simulink model "HHP_simulation"  (R2024b)
settings: Solver=ode23s  StartTime=0.0  StopTime=31104000  FixedStep=10  RelTol=2.42524E-1
undefined symbols (not defined in the file or in its folder): Ar, Br, c1, c33, c4, Cd, Cdl, Cr, Cu, Dd, DiameterLastPiece, dl, Dr, Du, gfunction, L1, L10, np, path_carnot, r_Trichter, Rechenradius, T_null, t_start, t_Trichter, Tdown_0, Tearth_anf, Temperature, Tup_0
libraries: carnot x3
settings Model: SimulationMode=accelerator  Creator=mdraihan  LastModifiedBy=mdraihan
settings SolverCC: MaxConsecutiveMinStep=50  SolverJacobianMethodControl=FullPerturbation  ShapePreserveControl=EnableAll  ZeroCrossControl=DisableAll
settings DataIOCC: LimitDataPoints=on  MaxDataPoints=100  SaveFinalState=on  SaveOperatingPoint=on  SaveFormat=Structure  ReturnWorkspaceOutputs=off  LoggingFileName=logsout
settings DebuggingCC: AlgebraicLoopMsg=none
settings RTWCC: GPUComputeCapability=3.5

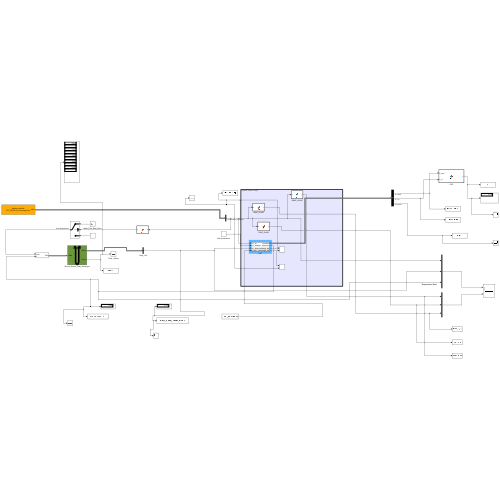
[thumbnail: Simulink's stored preview of the top-level diagram]
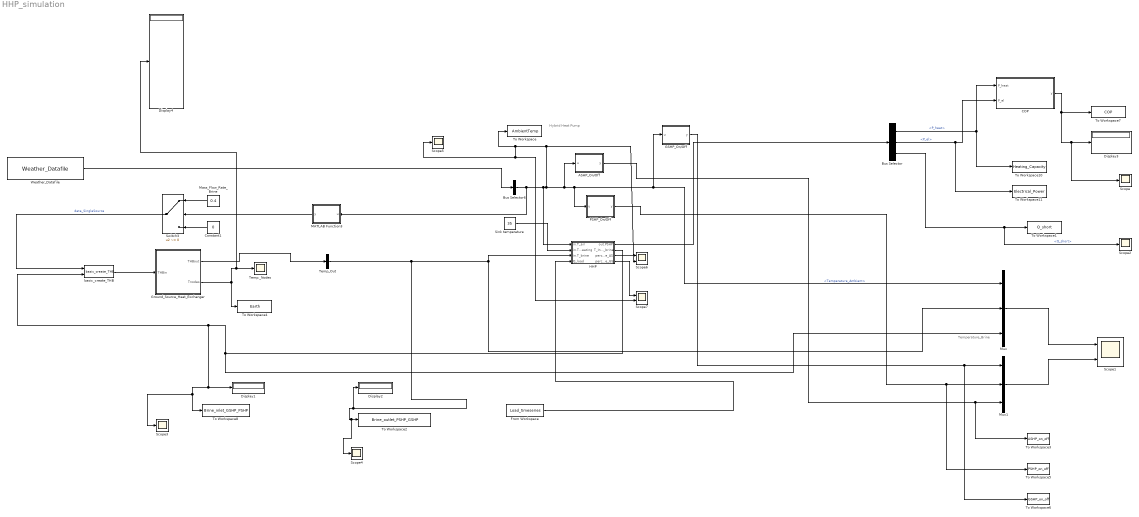
== system HHP_simulation ==
  note: Temperature_Brine
  note: Hybrid Heat Pump
  ASHP_On/Off : MATLAB Function  TreatAsAtomicUnit=on
  Bus Selector : BusSelector  OutputSignals=P_heat,P_el,Q_short
  Bus Selector6 : BusSelector  OutputSignals=Temperature_Ambient
  COP : MATLAB Function  TreatAsAtomicUnit=on
  Constant1 : Constant  Value=0
  Display{1..4} (4 alike) : Display
  From Workspace : FromWorkspace  VariableName=Load_timeseries
  GSHP_On/Off : MATLAB Function  TreatAsAtomicUnit=on
  Ground_Source_Heat_Exchanger : Subsystem  AncestorBlock=carnot/Source/Heat_Exchanger/Ground_Source_Heat_Exchanger  mask(ground source heat exchanger with variable massflow){Jahresmitteltemp_C=10, TGrad=0.025, lambdaErde=2.5, cpErde=1000, rhoErde=2200, lambdaFill=0.81, cpFill=3040, rhoFill=1180, lambda_Sondenrohr=0.48, Massenstrom=0.4, Sondenlaenge=70, B_sondenabstand=5, Sondendurchmesser=0.032, Bohrdurchmesser=0.12, Bu_param=0.12-0.032, Wanddicke_Sondenrohr=0.003, SondenFall=1 probe, DimVert=5, DimRad=10, Gitterfaktor=2.5, LastYear=0, qdot_precalc=10, show=off}
      mask prompts: Jahresmitteltemp_C "Average annual outdoor temperature  in °C"; TGrad "Temperature gradient in K/m, typical 0.025..0.04"; lambdaErde "Thermal conductivity ground in W/m/K"; cpErde "Heat capacity of the ground in J/kg/K"; rhoErde "Denstiy of the ground in kg/m³"; lambdaFill "Thermal conductivity filling in W/m/K"; cpFill "Heat capacity of the filling in J/kg/K"; rhoFill "Denstiy of the filling in kg/m³"; lambda_Sondenrohr "Thermal conductivity of pipe material  in W/m/K"; Massenstrom "Massflow in all ground probes in kg/s"; Sondenlaenge "H: Length of earth probe in m"; B_sondenabstand "B: Probe distance in m (= calculation diameter for single probe)"; Sondendurchmesser "Outer diameter of tube in m"; Bohrdurchmesser "Diameter of drilled hole in m"; Bu_param "Shank spacing in m (must be < borehole diameter)"; Wanddicke_Sondenrohr "Thickness of pipe wall in m"; SondenFall "Field geometry"; DimVert "No. of vertical nodes (typical 5, minimum 2)"; DimRad "No. of horizontal (radial) nodes (typical 10, minimum 3)"; Gitterfaktor "grid factor (typical 2.5, must be > 1)"; LastYear "Year (no precalculation = 0; steady state = 50)"; qdot_precalc "Extraction power per length in W/m (positive for heat removal)"; show "Display start conditions"
      mask help:
      | The CARNOT EWS model is a transient model for dynamic simulation of borehole heat exchangers or so-called vertical ground heat exchangers. The pipe model is for a double U-tube ground probe.  The model is based on the equations described by [Huber] and has been implemented using the state space model of Matlab/Simulink [Bianchi].
      | In the model the matrices are calculated for every timestep to take a variable massflow into account.
      |  See <Help> for literature.
      mask init:
      | DimAxi = max(DimVert*2,4);
      | DimRad = max(DimRad,3);
      | 
      | [Ad,Bd,Cd,Dd, Au,Bu,Cu,Du, Ad0,Bd0, Au0,Bu0, ...
      |     Ar,Br,Cr,Dr, Cdl, c1, c3, c31, c33, c4, c41, c5, c6, ...
      |     L1, L2, L10, L20, dl, Rechenradius, np, ...
      |     Tearth_anf, T_null, teta_fluid_ini, Tdown_0, Tup_0, ...
      |     Ts_Trichter, t_Trichter, r_Trichter, gfunction, t_start ...
      | ] = ...
      | CarnotCallbacks_EWS(LastYear, Massenstrom, qdot_precalc, ...
      |     SondenFall, B_sondenabstand, Sondenlaenge, Sondendurchmesser, ...
      |     Bohrdurchmesser, Bu_param, Wanddicke_Sondenrohr, ...
      |     Jahresmitteltemp_C, TGrad, ...
      |     lambdaErde, rhoErde, cpErde, ...
      |     lambdaFill, cpFill, rhoFill, lambda_Sondenrohr, ...
      |     DimAxi, DimRad, Gitterfaktor, show);
      mask Help: web(fullfile(path_carnot('help'),'Ground_Source_Heat_Exchanger.html'),'-helpbrowser')
      mask TypeOptions SondenFall: 1 probe | 2 probes B/H = 0.1 | 2 probes B/H = 0.05 | 3x6 probes B/H = 0.1 | 5x10 probes B/H = 0.1
      mask DialogControl ParameterTabVar0 Prompt: Thermal
      mask DialogControl ParameterTabVar01 Prompt: Geometry
      mask DialogControl ParameterTabVar012 Prompt: Calculation
      mask DialogControl Container6 Prompt: Precalculation of the ground temperature
      mask Display:
      | plot(0,10,100,90,[70,30],[80,80], ...
      |     [35,35,43,43,47,52,57,57,66,66,60,60,54,46,40,40,35], ...
      |     [84,87,87,20,13,13,21,87,87,84,84,20,10,10,20,84,84])
  HHP : Subsystem
  MATLAB Function3 : MATLAB Function  TreatAsAtomicUnit=on
  Mass_Flow_Rate_Brine : Constant  Value=0.4
  Mux : Mux  Inputs=3
  Mux1 : Mux  Inputs=3
  PSHP_On/Off : MATLAB Function  TreatAsAtomicUnit=on
  Scope{,2..5} (5 alike) : Scope
  Scope1 : Scope  NumInputPorts=2
  Scope6 : Scope  NumInputPorts=2
  Scope7 : Scope  NumInputPorts=2
  Sink temperature : Constant  Value=35
  Switch3 : Switch  Criteria=u2 ~= 0  SaturateOnIntegerOverflow=off
  Temp._Nodes : Scope
  Temp_Out : BusSelector  OutputSignals=Temperature  OutputAsBus=on
  To Workspace : ToWorkspace  VariableName=AmbientTemp  SaveFormat=Structure With Time  SampleTime=-1
  To Workspace1 : ToWorkspace  VariableName=Q_short  SaveFormat=Structure With Time  SampleTime=-1
  To Workspace10 : ToWorkspace  VariableName=Heating_Capacity  SaveFormat=Structure With Time  SampleTime=-1
  To Workspace11 : ToWorkspace  VariableName=Electrical_Power  SaveFormat=Structure With Time  SampleTime=-1
  To Workspace2 : ToWorkspace  VariableName=Brine_outlet_PSHP_GSHP  SaveFormat=Structure With Time  SampleTime=-1
      settings: Save2DSignal=2-D array (concatenate along first dimension)
  To Workspace3 : ToWorkspace  VariableName=ASHP_on_off  SaveFormat=Timeseries  SampleTime=-1
  To Workspace4 : ToWorkspace  VariableName=Earth  SaveFormat=Structure With Time  SampleTime=-1
      settings: Save2DSignal=2-D array (concatenate along first dimension)
  To Workspace5 : ToWorkspace  VariableName=PSHP_on_off  SaveFormat=Timeseries  SampleTime=-1
  To Workspace6 : ToWorkspace  VariableName=GSHP_on_off  SaveFormat=Timeseries  SampleTime=-1
  To Workspace7 : ToWorkspace  VariableName=COP  SampleTime=-1
      settings: Save2DSignal=2-D array (concatenate along first dimension)
  To Workspace8 : ToWorkspace  VariableName=Brine_inlet_GSHP_PSHP  SaveFormat=Structure With Time  SampleTime=-1
  Weather_Datafile : carnot/Weather/Weather_Datafile  PathName=path_carnot('data')  FileName='DE_TRY2010_04_averageYear.mat'  UserParam=off  VariableName=DE_TRY2010_04_averageYear  t_sample=3600
      settings: SourceProductName=Carnot
  basic_create_THB : carnot/Basic/Hydraulics/basic_create_THB  p=2e5  fluid=Water  mix=0  mix2=0  mix3=0  dia=0.03  hgt=0  mID=No Pressure Drop
      settings: SourceProductName=Carnot
  wires:
  Bus Selector/2 -> To Workspace11/1, COP/2(P_el)  "<P_el>"
  HHP/1(out.PSHP) -> Bus Selector/1
  Bus Selector/1 -> COP/1(P_heat), To Workspace10/1  "<P_heat>"
  Switch3/1 -> basic_create_THB/1  "data_SingleSource"
  Bus Selector6/1 -> Scope5/1, Scope7/2, To Workspace/1, Scope6/2, ASHP_On/Off/1(u), PSHP_On/Off/1(u), Mux/1, GSHP_On/Off/1(u), HHP/1(in.T_air), MATLAB Function3/1(u)  "<Temperature_Ambient>"
  Ground_Source_Heat_Exchanger/1(THBout) -> Temp_Out/1
  MATLAB Function3/1(y) -> Switch3/2
  Mass_Flow_Rate_Brine/1 -> Switch3/1
  GSHP_On/Off/1(y) -> To Workspace6/1, Mux1/1
  Mux/1 -> Scope1/1
  Sink temperature/1 -> HHP/2(in.T_heating)
  Weather_Datafile/1 -> Bus Selector6/1
  Constant1/1 -> Switch3/3
  HHP/2(T_Inlet_brine) -> Scope3/1, To Workspace8/1, Display1/1, basic_create_THB/2, Mux/3
  basic_create_THB/1 -> Ground_Source_Heat_Exchanger/1(THBin)
  Ground_Source_Heat_Exchanger/2(Tnodes) -> To Workspace4/1, Temp._Nodes/1, Display4/1
  COP/1(y) -> To Workspace7/1, Scope/1, Display3/1
  ASHP_On/Off/1(y) -> To Workspace3/1, Mux1/3
  From Workspace/1 -> HHP/4(Q_load)
  Mux1/1 -> Scope1/2
  Bus Selector/3 -> Scope2/1, To Workspace1/1  "<Q_short>"
  Temp_Out/1 -> Display2/1, Scope4/1, To Workspace2/1, Mux/2, HHP/3(in.T_brine)
  PSHP_On/Off/1(y) -> To Workspace5/1, Mux1/2
  HHP/3(percentage_AS) -> Scope6/1
  HHP/4(percentage_GS) -> Scope7/1

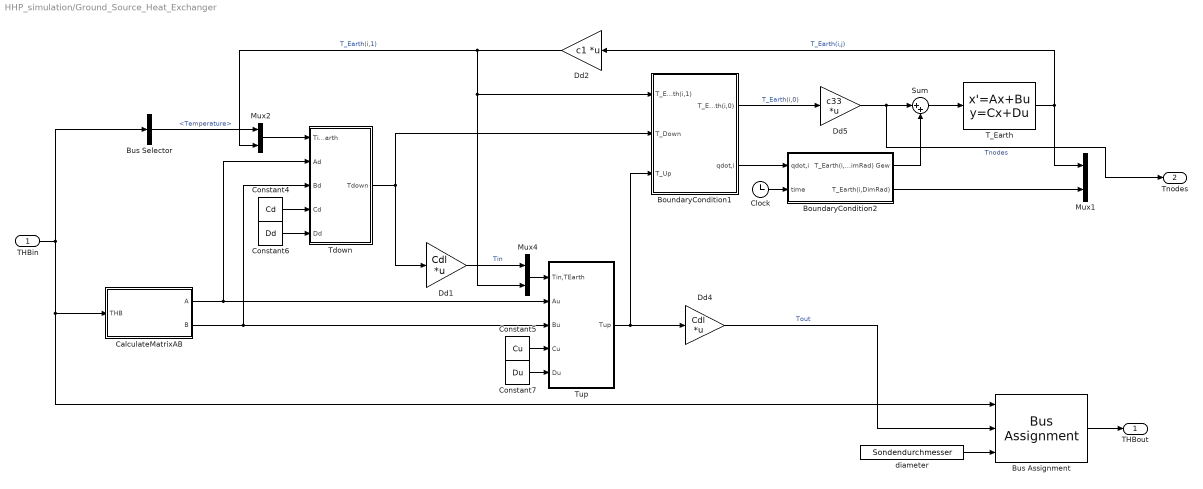
== system HHP_simulation/Ground_Source_Heat_Exchanger ==
  THBin : Inport
  BoundaryCondition1 : Subsystem
  BoundaryCondition2 : Subsystem
  Bus Assignment : BusAssignment  AssignedSignals=Temperature,DiameterLastPiece
  Bus Selector : BusSelector  OutputSignals=Temperature
  CalculateMatrixAB : Subsystem
  Clock : Clock
  Constant4 : Constant  Value=Cd
  Constant5 : Constant  Value=Cu
  Constant6 : Constant  Value=Dd
  Constant7 : Constant  Value=Du
  Dd1 : Gain  Gain=Cdl  Multiplication=Matrix(K*u)  SaturateOnIntegerOverflow=on  OutDataTypeStr=Inherit: Same as input  ParamDataTypeStr=Inherit: Same as input
  Dd2 : Gain  Gain=c1  Multiplication=Matrix(K*u)  SaturateOnIntegerOverflow=on  OutDataTypeStr=Inherit: Same as input  ParamDataTypeStr=Inherit: Same as input
  Dd4 : Gain  Gain=Cdl  Multiplication=Matrix(K*u) (u vector)  SaturateOnIntegerOverflow=on  OutDataTypeStr=Inherit: Same as input  ParamDataTypeStr=Inherit: Same as input
  Dd5 : Gain  Gain=c33  Multiplication=Matrix(K*u) (u vector)  SaturateOnIntegerOverflow=on  OutDataTypeStr=Inherit: Same as input  ParamDataTypeStr=Inherit: Same as input
  Mux1 : Mux  Inputs=2
  Mux2 : Mux  Inputs=2
  Mux4 : Mux  Inputs=2
  Sum : Sum  Inputs=|++  InputSameDT=on  SaturateOnIntegerOverflow=on  OutDataTypeStr=Inherit: Same as first input
  T_Earth : StateSpace  A=Ar  B=Br  C=Cr  D=Dr  InitialCondition=Tearth_anf(:)
  Tdown : Subsystem
  Tup : Subsystem
  diameter : Constant  Value=Sondendurchmesser
  THBout : Outport  VectorParamsAs1DForOutWhenUnconnected=off
  Tnodes : Outport  Port=2  VectorParamsAs1DForOutWhenUnconnected=off
  wires:
  CalculateMatrixAB/2(B) -> Tup/3(Bu), Tdown/3(Bd)
  CalculateMatrixAB/1(A) -> Tup/2(Au), Tdown/2(Ad)
  BoundaryCondition1/2(qdot,i) -> BoundaryCondition2/1(qdot,i)
  Dd4/1 -> Bus Assignment/2  "Tout"
  Bus Assignment/1 -> THBout/1
  diameter/1 -> Bus Assignment/3
  THBin/1 -> CalculateMatrixAB/1(THB), Bus Assignment/1, Bus Selector/1
  BoundaryCondition2/2(T_Earth(i,DimRad)) -> Mux1/2
  Dd2/1 -> Mux4/2, BoundaryCondition1/1(T_Earth(i,1)), Mux2/2  "T_Earth(i,1)"
  BoundaryCondition1/1(T_Earth(i,0)) -> Dd5/1  "T_Earth(i,0)"
  Sum/1 -> T_Earth/1
  BoundaryCondition2/1(T_Earth(i,DimRad) Gew) -> Sum/2
  Tup/1(Tup) -> Dd4/1, BoundaryCondition1/3(T_Up)
  T_Earth/1 -> Dd2/1, Mux1/1  "T_Earth(i,j)"
  Dd1/1 -> Mux4/1  "Tin"
  Mux4/1 -> Tup/1(Tin,TEarth)
  Mux2/1 -> Tdown/1(Tin,TEarth)
  Tdown/1(Tdown) -> Dd1/1, BoundaryCondition1/2(T_Down)
  Constant4/1 -> Tdown/4(Cd)
  Constant6/1 -> Tdown/5(Dd)
  Constant7/1 -> Tup/5(Du)
  Constant5/1 -> Tup/4(Cu)
  Bus Selector/1 -> Mux2/1  "<Temperature>"
  Clock/1 -> BoundaryCondition2/2(time)
  Dd5/1 -> Tnodes/1, Sum/1  "Tnodes"

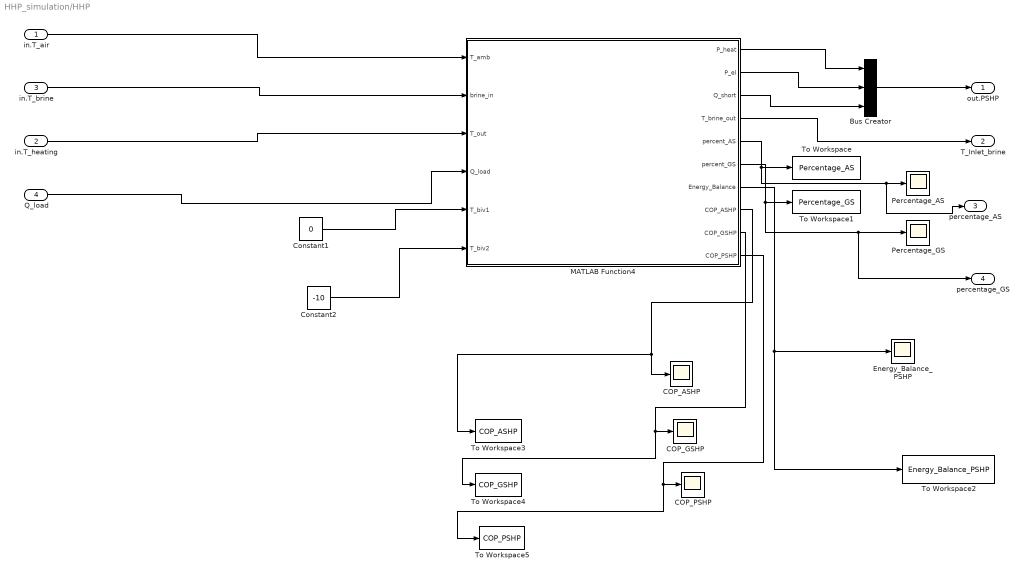
== system HHP_simulation/HHP ==
  in.T_air : Inport
  in.T_heating : Inport  Port=2
  in.T_brine : Inport  Port=3
  Q_load : Inport  Port=4
  Bus Creator : BusCreator  Inputs=3
  COP_ASHP : Scope
  COP_GSHP : Scope
  COP_PSHP : Scope
  Constant1 : Constant  Value=0
  Constant2 : Constant  Value=-10
  Energy_Balance_PSHP : Scope
  MATLAB Function4 : MATLAB Function  TreatAsAtomicUnit=on
  Percentage_AS : Scope
  Percentage_GS : Scope
  To Workspace : ToWorkspace  VariableName=Percentage_AS  SaveFormat=Structure  SampleTime=-1
  To Workspace1 : ToWorkspace  VariableName=Percentage_GS  SaveFormat=Structure  SampleTime=-1
  To Workspace2 : ToWorkspace  VariableName=Energy_Balance_PSHP  SaveFormat=Structure  SampleTime=-1
  To Workspace3 : ToWorkspace  VariableName=COP_ASHP  SaveFormat=Structure  SampleTime=-1
  To Workspace4 : ToWorkspace  VariableName=COP_GSHP  SaveFormat=Structure  SampleTime=-1
  To Workspace5 : ToWorkspace  VariableName=COP_PSHP  SaveFormat=Structure  SampleTime=-1
  out.PSHP : Outport
  T_Inlet_brine : Outport  Port=2
  percentage_AS : Outport  Port=3
  percentage_GS : Outport  Port=4
  wires:
  in.T_air/1 -> MATLAB Function4/1(T_amb)
  in.T_heating/1 -> MATLAB Function4/3(T_out)
  in.T_brine/1 -> MATLAB Function4/2(brine_in)
  Q_load/1 -> MATLAB Function4/4(Q_load)
  MATLAB Function4/4(T_brine_out) -> T_Inlet_brine/1
  MATLAB Function4/2(P_el) -> Bus Creator/2
  MATLAB Function4/1(P_heat) -> Bus Creator/1
  MATLAB Function4/3(Q_short) -> Bus Creator/3
  Bus Creator/1 -> out.PSHP/1
  MATLAB Function4/5(percent_AS) -> percentage_AS/1, Percentage_AS/1, To Workspace/1
  MATLAB Function4/6(percent_GS) -> percentage_GS/1, Percentage_GS/1, To Workspace1/1
  MATLAB Function4/7(Energy_Balance) -> To Workspace2/1, Energy_Balance_PSHP/1
  MATLAB Function4/8(COP_ASHP) -> To Workspace3/1, COP_ASHP/1
  MATLAB Function4/9(COP_GSHP) -> To Workspace4/1, COP_GSHP/1
  MATLAB Function4/10(COP_PSHP) -> To Workspace5/1, COP_PSHP/1
  Constant1/1 -> MATLAB Function4/5(T_biv1)
  Constant2/1 -> MATLAB Function4/6(T_biv2)

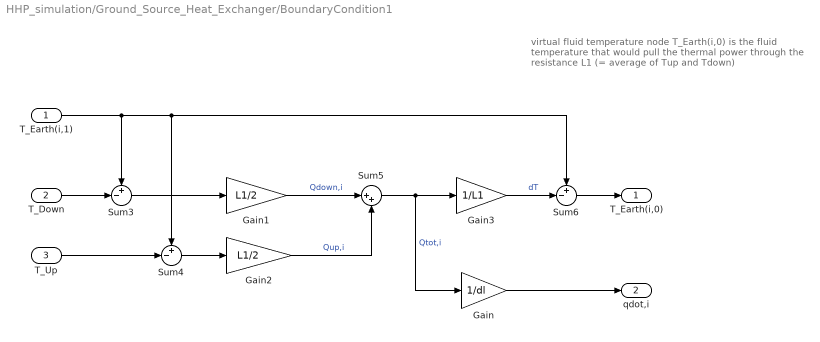
== system HHP_simulation/Ground_Source_Heat_Exchanger/BoundaryCondition1 ==
  note: virtual fluid temperature node T_Earth(i,0) is the
      | fluid temperature that would pull the thermal
      | power through the resistance L1 (= average of
      | Tup and Tdown)
  T_Earth(i,1) : Inport
  T_Down : Inport  Port=2
  T_Up : Inport  Port=3
  Gain : Gain  Gain=1/dl
  Gain1 : Gain  Gain=L1/2  SaturateOnIntegerOverflow=on  OutDataTypeStr=Inherit: Same as input  ParamDataTypeStr=Inherit: Same as input
  Gain2 : Gain  Gain=L1/2  SaturateOnIntegerOverflow=on  OutDataTypeStr=Inherit: Same as input  ParamDataTypeStr=Inherit: Same as input
  Gain3 : Gain  Gain=1/L1  SaturateOnIntegerOverflow=on  OutDataTypeStr=Inherit: Same as input  ParamDataTypeStr=Inherit: Same as input
  Sum3 : Sum  Inputs=+-|  InputSameDT=on  SaturateOnIntegerOverflow=on  OutDataTypeStr=Inherit: Same as first input
  Sum4 : Sum  Inputs=+-|  InputSameDT=on  SaturateOnIntegerOverflow=on  OutDataTypeStr=Inherit: Same as first input
  Sum5 : Sum  Inputs=|++  InputSameDT=on  SaturateOnIntegerOverflow=on  OutDataTypeStr=Inherit: Same as first input
  Sum6 : Sum  Inputs=+-|  InputSameDT=on  SaturateOnIntegerOverflow=on  OutDataTypeStr=Inherit: Same as first input
  T_Earth(i,0) : Outport  VectorParamsAs1DForOutWhenUnconnected=off
  qdot,i : Outport  Port=2  VectorParamsAs1DForOutWhenUnconnected=off
  wires:
  Gain/1 -> qdot,i/1
  Sum6/1 -> T_Earth(i,0)/1
  T_Earth(i,1)/1 -> Sum6/1, Sum4/1, Sum3/1
  Gain3/1 -> Sum6/2  "dT"
  Sum5/1 -> Gain/1, Gain3/1  "Qtot,i"
  Gain2/1 -> Sum5/2  "Qup,i"
  Gain1/1 -> Sum5/1  "Qdown,i"
  Sum4/1 -> Gain2/1
  Sum3/1 -> Gain1/1
  T_Down/1 -> Sum3/2
  T_Up/1 -> Sum4/2

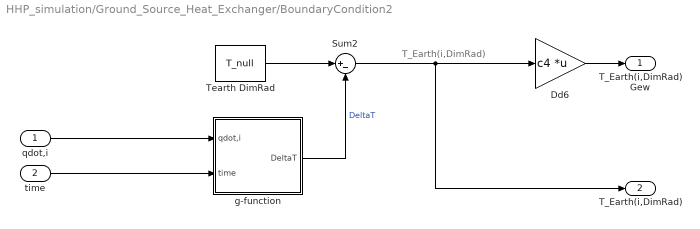
== system HHP_simulation/Ground_Source_Heat_Exchanger/BoundaryCondition2 ==
  note: T_Earth(i,DimRad)
  qdot,i : Inport
  time : Inport  Port=2
  Dd6 : Gain  Gain=c4  Multiplication=Matrix(K*u)  SaturateOnIntegerOverflow=on  OutDataTypeStr=Inherit: Same as input  ParamDataTypeStr=Inherit: Same as input
  Sum2 : Sum  Inputs=|+-  InputSameDT=on  SaturateOnIntegerOverflow=on  OutDataTypeStr=Inherit: Same as first input
  Tearth DimRad : Constant  Value=T_null  VectorParams1D=off
  g-function : Subsystem
  T_Earth(i,DimRad) Gew : Outport  VectorParamsAs1DForOutWhenUnconnected=off
  T_Earth(i,DimRad) : Outport  Port=2  VectorParamsAs1DForOutWhenUnconnected=off
  wires:
  Sum2/1 -> Dd6/1, T_Earth(i,DimRad)/1
  Tearth DimRad/1 -> Sum2/1
  qdot,i/1 -> g-function/1(qdot,i)
  Dd6/1 -> T_Earth(i,DimRad) Gew/1
  g-function/1(DeltaT) -> Sum2/2  "DeltaT"
  time/1 -> g-function/2(time)

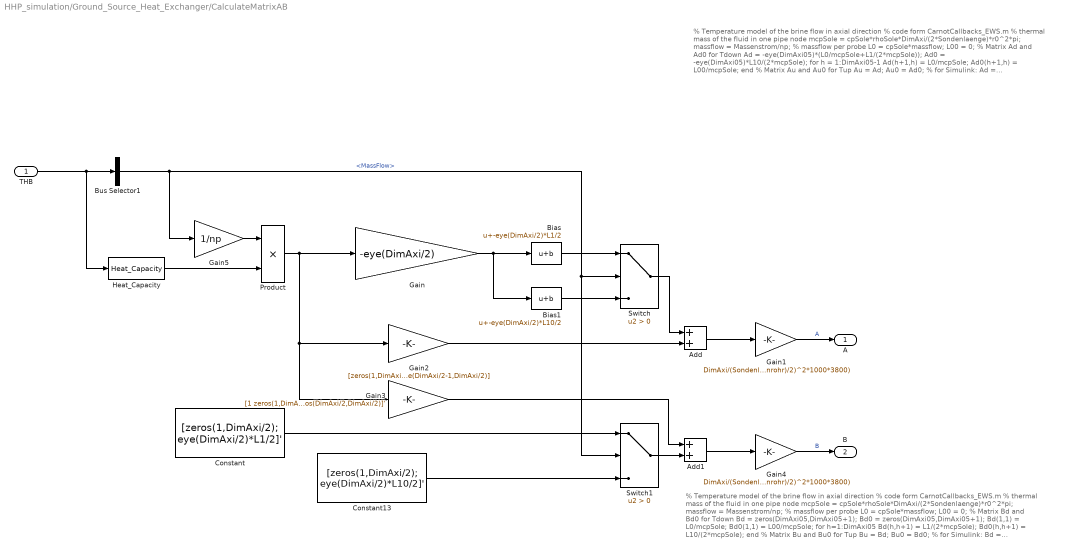
== system HHP_simulation/Ground_Source_Heat_Exchanger/CalculateMatrixAB ==
  note: % Temperature model of the brine flow in axial direction
      | % code form CarnotCallbacks_EWS.m
      | % thermal mass of the fluid in one pipe node
      | mcpSole = cpSole*rhoSole*DimAxi/(2*Sondenlaenge)*r0^2*pi;
      | massflow = Massenstrom/np; % massflow per probe
      | L0 = cpSole*massflow;
      | L00 = 0;
      | % Matrix Bd and Bd0 for Tdown
      | Bd = zeros(DimAxi05,DimAxi05+1);
      | Bd0 = zeros(DimAxi05,DimAxi05+1);
      | Bd(1,1) = L0/mcpSole;
      | Bd0(1,1) = L00/mcpSole;
      | for h=1:DimAxi05
      | Bd(h,h+1) = L1/(2*mcpSole);
      | Bd0(h,h+1) = L10/(2*mcpSole);
      | end
      | % Matrix Bu and Bu0 for Tup
      | Bu = Bd;
      | Bu0 = Bd0;
      |
      | % for Simulink:
      | Bd = [zeros(1,DimAxi/2); eye(DimAxi/2)*L1/2]'
      | Bd = Bd + [1 zeros(1,DimAxi/2-1); zeros(DimAxi/2,DimAxi/2)]'
      | Bd = Bd * DimAxi / ...
      | (Sondenlaenge*2*pi*((Sondendurchmesser-Wanddicke_Sondenrohr)/2)^2*1000*3800)
  note: % Temperature model of the brine flow in axial direction
      | % code form CarnotCallbacks_EWS.m
      | % thermal mass of the fluid in one pipe node
      | mcpSole = cpSole*rhoSole*DimAxi/(2*Sondenlaenge)*r0^2*pi;
      | massflow = Massenstrom/np; % massflow per probe
      | L0 = cpSole*massflow;
      | L00 = 0;
      | % Matrix Ad and Ad0 for Tdown
      | Ad = -eye(DimAxi05)*(L0/mcpSole+L1/(2*mcpSole));
      | Ad0 = -eye(DimAxi05)*L10/(2*mcpSole);
      | for h = 1:DimAxi05-1
      | Ad(h+1,h) = L0/mcpSole;
      | Ad0(h+1,h) = L00/mcpSole;
      | end
      | % Matrix Au and Au0 for Tup
      | Au = Ad;
      | Au0 = Ad0;
      |
      | % for Simulink:
      | Ad = -eye(DimAxi05)
      | Ad = Ad - eye(DimAxi/2)*L1/2
      | Ad = Ad + [zeros(1,DimAxi/2); eye(DimAxi/2-1,DimAxi/2)]
      | Ad = Ad * DimAxi / ...
      | (Sondenlaenge*2*pi*((Sondendurchmesser-Wanddicke_Sondenrohr)/2)^2*1000*3800)
  THB : Inport
  Add : Sum
  Add1 : Sum
  Bias : Bias  Bias=-eye(DimAxi/2)*L1/2  SaturateOnIntegerOverflow=off
  Bias1 : Bias  Bias=-eye(DimAxi/2)*L10/2  SaturateOnIntegerOverflow=off
  Bus Selector1 : BusSelector  OutputSignals=MassFlow
  Constant : Constant  Value=[zeros(1,DimAxi/2); eye(DimAxi/2)*L1/2]'  VectorParams1D=off
  Constant13 : Constant  Value=[zeros(1,DimAxi/2); eye(DimAxi/2)*L10/2]'  VectorParams1D=off
  Gain : Gain  Gain=-eye(DimAxi/2)
  Gain1 : Gain  Gain=DimAxi/(Sondenlaenge*2*pi*((Sondendurchmesser-Wanddicke_Sondenrohr)/2)^2*1000*3800)
  Gain2 : Gain  Gain=[zeros(1,DimAxi/2); eye(DimAxi/2-1,DimAxi/2)]
  Gain3 : Gain  Gain=[1 zeros(1,DimAxi/2-1); zeros(DimAxi/2,DimAxi/2)]'
  Gain4 : Gain  Gain=DimAxi/(Sondenlaenge*2*pi*((Sondendurchmesser-Wanddicke_Sondenrohr)/2)^2*1000*3800)
  Gain5 : Gain  Gain=1/np
  Heat_Capacity : carnot/Basic/Material_Properties/Heat_Capacity  VariantControl=CarlibClassic  INPUTARGUMENTS=THB  DEBUGLEVEL=DEBUGLEVEL  MAXTOTALWARNINGS=0  MAXCONSECUTIVEWARNINGS=0  WRITETOFILE=0  FILENAME='errors.txt'
      settings: SourceProductName=Carnot
  Product : Product
  Switch : Switch  Criteria=u2 > Threshold  SaturateOnIntegerOverflow=off  InputSameDT=off
  Switch1 : Switch  Criteria=u2 > Threshold  SaturateOnIntegerOverflow=off  InputSameDT=off
  A : Outport
  B : Outport  Port=2
  wires:
  Gain5/1 -> Product/1
  Gain4/1 -> B/1  "B"
  Gain1/1 -> A/1  "A"
  Gain3/1 -> Add1/1
  Add1/1 -> Gain4/1
  Constant/1 -> Switch1/1
  Heat_Capacity/1 -> Product/2
  Gain2/1 -> Add/2
  Switch/1 -> Add/1
  Constant13/1 -> Switch1/3
  Add/1 -> Gain1/1
  Switch1/1 -> Add1/2
  Bias/1 -> Switch/1
  Product/1 -> Gain/1, Gain2/1, Gain3/1
  Bias1/1 -> Switch/3
  Gain/1 -> Bias/1, Bias1/1
  Bus Selector1/1 -> Gain5/1, Switch1/2, Switch/2  "<MassFlow>"
  THB/1 -> Heat_Capacity/1, Bus Selector1/1

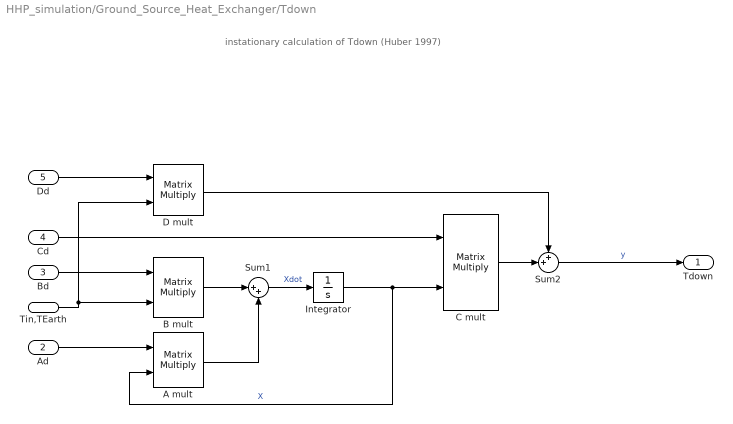
== system HHP_simulation/Ground_Source_Heat_Exchanger/Tdown ==
  note: instationary calculation of Tdown (Huber 1997)
  Tin,TEarth : Inport
  Ad : Inport  Port=2
  Bd : Inport  Port=3
  Cd : Inport  Port=4
  Dd : Inport  Port=5
  A mult : Product  Multiplication=Matrix(*)  RndMeth=Zero
  B mult : Product  Multiplication=Matrix(*)  RndMeth=Zero
  C mult : Product  Multiplication=Matrix(*)  RndMeth=Zero
  D mult : Product  Multiplication=Matrix(*)  RndMeth=Zero
  Integrator : Integrator  InitialCondition=Tdown_0
  Sum1 : Sum  Inputs=|++
  Sum2 : Sum  Inputs=++|
  Tdown : Outport  VectorParamsAs1DForOutWhenUnconnected=off
  wires:
  Sum2/1 -> Tdown/1  "y"
  Tin,TEarth/1 -> B mult/2, D mult/2
  D mult/1 -> Sum2/1
  C mult/1 -> Sum2/2
  B mult/1 -> Sum1/1
  Sum1/1 -> Integrator/1  "Xdot"
  Integrator/1 -> C mult/2, A mult/2  "X"
  A mult/1 -> Sum1/2
  Ad/1 -> A mult/1
  Cd/1 -> C mult/1
  Dd/1 -> D mult/1
  Bd/1 -> B mult/1

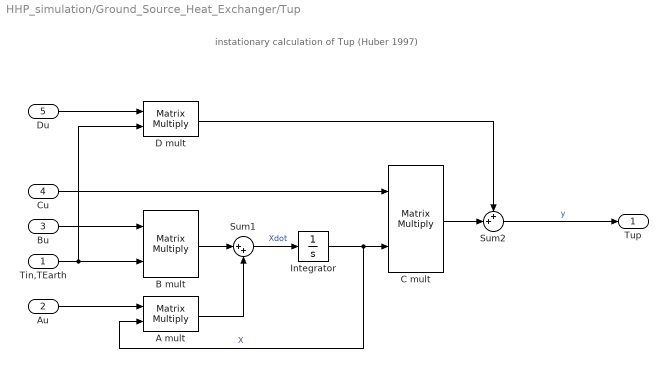
== system HHP_simulation/Ground_Source_Heat_Exchanger/Tup ==
  note: instationary calculation of Tup (Huber 1997)
  Tin,TEarth : Inport
  Au : Inport  Port=2
  Bu : Inport  Port=3
  Cu : Inport  Port=4
  Du : Inport  Port=5
  A mult : Product  Multiplication=Matrix(*)  RndMeth=Zero
  B mult : Product  Multiplication=Matrix(*)  RndMeth=Zero
  C mult : Product  Multiplication=Matrix(*)  RndMeth=Zero
  D mult : Product  Multiplication=Matrix(*)  RndMeth=Zero
  Integrator : Integrator  InitialCondition=Tup_0
  Sum1 : Sum  Inputs=|++
  Sum2 : Sum  Inputs=++|
  Tup : Outport  VectorParamsAs1DForOutWhenUnconnected=off
  wires:
  Sum2/1 -> Tup/1  "y"
  Tin,TEarth/1 -> D mult/2, B mult/2
  D mult/1 -> Sum2/1
  C mult/1 -> Sum2/2
  B mult/1 -> Sum1/1
  Sum1/1 -> Integrator/1  "Xdot"
  Integrator/1 -> A mult/2, C mult/2  "X"
  A mult/1 -> Sum1/2
  Bu/1 -> B mult/1
  Au/1 -> A mult/1
  Cu/1 -> C mult/1
  Du/1 -> D mult/1

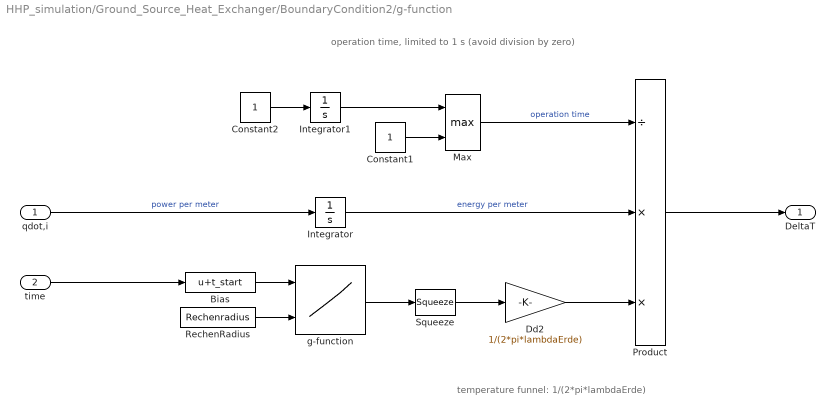
== system HHP_simulation/Ground_Source_Heat_Exchanger/BoundaryCondition2/g-function ==
  note: temperature funnel: 1/(2*pi*lambdaErde)
  note: operation time, limited to 1 s (avoid division by zero)
  qdot,i : Inport
  time : Inport  Port=2
  Bias : Bias  Bias=t_start  SaturateOnIntegerOverflow=off
  Constant1 : Constant
  Constant2 : Constant
  Dd2 : Gain  Gain=1/(2*pi*lambdaErde)  SaturateOnIntegerOverflow=on  OutDataTypeStr=Inherit: Same as input  ParamDataTypeStr=Inherit: Same as input
  Integrator : Integrator
  Integrator1 : Integrator  LowerSaturationLimit=1
  Max : MinMax  Function=max  Inputs=2
  Product : Product  Inputs=/**  InputSameDT=on  RndMeth=Zero  SaturateOnIntegerOverflow=on  OutDataTypeStr=Inherit: Same as first input
  RechenRadius : Constant  Value=Rechenradius  VectorParams1D=off
  Squeeze : Squeeze
  g-function : Lookup_n-D  BreakpointsForDimension1=t_Trichter  BreakpointsForDimension2=r_Trichter  BeginIndexSearchUsingPreviousIndexResult=on  Table=gfunction  InternalRulePriority=Speed  RndMeth=Simplest
      settings: InputPortMap=u0,u1
  DeltaT : Outport  VectorParamsAs1DForOutWhenUnconnected=off
  wires:
  Bias/1 -> g-function/1
  time/1 -> Bias/1
  Constant2/1 -> Integrator1/1
  Max/1 -> Product/1  "operation time"
  Constant1/1 -> Max/2
  Integrator1/1 -> Max/1
  Integrator/1 -> Product/2  "energy per meter"
  Squeeze/1 -> Dd2/1
  qdot,i/1 -> Integrator/1  "power per meter"
  g-function/1 -> Squeeze/1
  Product/1 -> DeltaT/1
  Dd2/1 -> Product/3
  RechenRadius/1 -> g-function/2

== matlab function HHP_simulation/ASHP_On//Off ==
  data: u input; y output
function y = fcn(u)
    % Function to check if the temperature is between 5°C and 13°C
    % Inputs:
    %   u - Temperature (numeric or part of a structure)
    % Outputs:
    %   y - 1 if the temperature is between 5°C and 13°C, 0 otherwise

    % Initialize output
    y = 0;

    % Define the field name (update this if necessary)
    fieldName = 'Temp';

    % Check if input is numeric
    if isnumeric(u)
        % Main logic: check if within range
        if u >= 5 && u <= 13
            y = 1;
        end
    % Check if input is a structure
    elseif isstruct(u)
        % Ensure the structure has the expected field
        if isfield(u, fieldName)
            temp = u.(fieldName); % Extract the temperature field

            % Ensure the extracted value is numeric
            if isnumeric(temp)
                % Main logic: check if within range
                if temp >= 5 && temp <= 13
                    y = 1;
                end
            else
                error('The field "%s" must contain numeric data.', fieldName);
            end
        else
            error('The input structure does not have the field "%s".', fieldName);
        end
    else
        % Handle unsupported input types
        error('Input must be either numeric or a structure with a numeric field "%s".', fieldName);
    end
end

== matlab function HHP_simulation/COP ==
  data: P_heat input; y output; P_el input
function y = fcn(P_heat, P_el)
    % Function to calculate COP based on heating capacity and electrical power.
    % If the heat pump is operating (both P_heat and P_el nonzero), the COP 
    % is computed as P_heat / P_el and forced to be at least 1.
    % If the heat pump is off (either input is 0), the COP is set to 0.
    %
    % Inputs:
    %   P_heat - Heating capacity of the heat pump (W)
    %   P_el   - Electrical power input to the heat pump (W)
    %
    % Outputs:
    %   y - Calculated COP (dimensionless)

    % Handle negative values by treating them as zero.
    if P_heat < 0
        P_heat = 0;
    end
    if P_el < 0
        P_el = 0;
    end

    % Check if the system is off (either P_heat or P_el is zero)
    if (P_heat == 0 || P_el == 0)
        y = 0; % Off condition
    else
        % Calculate COP normally.
        y = P_heat / P_el;
        % If COP is less than 1, set it to 1 (when operating, COP cannot be < 1).
        if y < 1
            y = 1;
        end
    end
end

== matlab function HHP_simulation/HHP/MATLAB Function4 ==
  data: T_amb input; P_heat output; brine_in input; T_out input; Q_load input; P_el output; Q_short output; T_brine_out output; percent_AS output; percent_GS output; Energy_Balance output; COP_ASHP output; COP_GSHP output; COP_PSHP output; T_biv1 input; T_biv2 input
function [P_heat, P_el, Q_short, T_brine_out, percent_AS, percent_GS, Energy_Balance, COP_ASHP, COP_GSHP, COP_PSHP] = hpHeatingPartLoad_Parallel_Final(...
        T_amb, brine_in, T_out, Q_load, T_biv1, T_biv2)
    
    NO_LOAD_THRESHOLD  = 1.0;
    T_amb              = double(T_amb(1));
    brine_in           = double(brine_in(1));
    T_out              = double(T_out(1));
    Q_load             = double(Q_load(1));
    
    if Q_load <= NO_LOAD_THRESHOLD
        P_heat=0; P_el=0; Q_short=Q_load; T_brine_out=brine_in; percent_AS=0;
        percent_GS=0; Energy_Balance=0; COP_ASHP=0; COP_GSHP=0; COP_PSHP=0;
        return;
    end
    
    if T_amb > T_biv1
        Q_AS = Q_load;
        Q_GS = 0;
    elseif T_amb >= T_biv2
        Q_AS = 0;
        Q_GS = Q_load;
    else
        ratio_base = min(max((T_biv2 - T_amb) / 10.0, 0), 1.0);
        ratio_GS = 0.7 + ratio_base * 0.2;
        ratio_AS = 1.0 - ratio_GS;
        Q_AS = Q_load * ratio_AS;
        Q_GS = Q_load * ratio_GS;
    end
    
    m_dot_GS = 0.4;
    delta_T = T_out - brine_in;
    if delta_T > 40, m_dot_GS = 0.6;
    elseif delta_T > 30, m_dot_GS = 0.5;
    else, m_dot_GS = 0.4; end
    if brine_in < 2, m_dot_GS = m_dot_GS * 1.25; end
    
    P_heat_AS=0; P_el_AS=0; Q_short_AS=0;
    P_heat_GS=0; P_el_GS=0; Q_short_GS=0; T_brine_out=brine_in;
    if Q_AS > 0
        [P_heat_AS, P_el_AS, Q_short_AS] = hpHeatingPartLoad_ASHP_Original_PLM(T_amb, T_out, Q_AS);
    end
    if Q_GS > 0
        [P_heat_GS, P_el_GS, Q_short_GS, T_brine_out] = ...
            hpHeatingPartLoad_GSHP_Original_PLM(brine_in, T_out, Q_GS, m_dot_GS);
    end
    
    P_heat  = P_heat_AS + P_heat_GS;
    P_el    = P_el_AS   + P_el_GS;
    Q_short = Q_short_AS + Q_short_GS;
    
    if Q_short > 0 && P_heat > 0
        base_cop = P_heat / P_el;
        stage_up_cop = base_cop * 0.97;
        max_additional_heat = P_heat * 0.15;
        
        P_heat_extra = min(Q_short, max_additional_heat);
        P_el_extra = 0;
        if stage_up_cop > 0
            P_el_extra = P_heat_extra / stage_up_cop;
        end

        P_heat = P_heat + P_heat_extra;
        P_el = P_el + P_el_extra;
        
        Q_short = max(0, Q_load - P_heat);
    end

    if (P_heat > 0) && (P_el > 0)
        if T_amb < T_biv2, max_allowed_COP = 5.0; 
        elseif T_amb > T_biv1, max_allowed_COP = 4.0;
        else, max_allowed_COP = 5.0; end
        current_COP = P_heat / P_el;
        transition_start = max_allowed_COP * 0.75;
        if current_COP > transition_start
            excess_COP = current_COP - transition_start;
            limiting_factor = 1.0 - exp(-3.0 * excess_COP / (max_allowed_COP - transition_start));
            max_excess_allowed = (max_allowed_COP - transition_start) * limiting_factor;
            target_COP = min(transition_start + max_excess_allowed, max_allowed_COP*0.999);
            P_el = P_heat / target_COP;
        end
    end
    
    percent_AS = 0; percent_GS = 0;
    if P_heat > 0
        P_heat_total_no_extra = P_heat_AS + P_heat_GS;
        if P_heat_total_no_extra > 0
             percent_AS = 100 * (P_heat_AS / P_heat_total_no_extra);
             percent_GS = 100 * (P_heat_GS / P_heat_total_no_extra);
        end
    end
    Energy_Balance = P_heat - P_el - ( (P_heat_AS-P_el_AS) + (P_heat_GS-P_el_GS) );

    COP_ASHP = 0; COP_GSHP = 0; COP_PSHP = 0;
    if (P_el > 0) && (P_heat > 0)
        total_COP = P_heat / P_el;
        if T_amb > T_biv1
            temp_range = T_biv1 - T_biv2;
            if temp_range <= 0, temp_range = 12; end
            temp_factor   = max(0.6, min(1.0, (T_amb - T_biv2) / temp_range));
            output_factor = max(0.7, min(1.0, 1 - (T_out - 30)/25 ));
            COP_ASHP = min(total_COP * (temp_factor * output_factor), 4.0 * 0.999);
        elseif T_amb >= T_biv2
            COP_GSHP = total_COP;
        else 
            COP_PSHP = total_COP;
        end
    end
end

function [P_heat, P_el, Q_short] = hpHeatingPartLoad_ASHP_Original_PLM(T_amb, T_out, Q_load)
    if (Q_load <= 0) || (T_amb < -20), P_heat = 0; P_el = 0; Q_short = Q_load; return; end
    T_amb_vec = [-15, -7, 2, 7, 12]; T_out_vec = [30, 35, 40, 45];
    CapacityMatrix = [ 2.47, 2.87, 3.27, 3.64, 4.00; 2.33, 2.73, 3.13, 3.49, 3.85; 2.18, 2.58, 2.98, 3.35, 3.71; 2.04, 2.44, 2.84, 3.20, 3.56 ];
    PowerMatrix = [ 1.20, 0.98, 0.84, 0.78, 0.74; 1.39, 1.14, 0.98, 0.90, 0.82; 1.57, 1.32, 1.07, 0.97, 0.90; 1.74, 1.50, 1.20, 1.12, 1.02 ];
    T_amb_lower_idx=1; for i=1:length(T_amb_vec), if T_amb>=T_amb_vec(i), T_amb_lower_idx=i; end, end
    if T_amb_lower_idx==length(T_amb_vec), T_amb_upper_idx=T_amb_lower_idx; else, T_amb_upper_idx=T_amb_lower_idx+1; end
    T_out_lower_idx=1; for i=1:length(T_out_vec), if T_out>=T_out_vec(i), T_out_lower_idx=i; end, end
    if T_out_lower_idx==length(T_out_vec), T_out_upper_idx=T_out_lower_idx; else, T_out_upper_idx=T_out_lower_idx+1; end
    if (T_amb_lower_idx==T_amb_upper_idx)||(T_out_lower_idx==T_out_upper_idx), Q_rated=CapacityMatrix(T_out_lower_idx,T_amb_lower_idx); P_rated=PowerMatrix(T_out_lower_idx,T_amb_lower_idx);
    else
        x1=T_amb_vec(T_amb_lower_idx);x2=T_amb_vec(T_amb_upper_idx);y1=T_out_vec(T_out_lower_idx);y2=T_out_vec(T_out_upper_idx);
        Q11=CapacityMatrix(T_out_lower_idx,T_amb_lower_idx);Q12=CapacityMatrix(T_out_upper_idx,T_amb_lower_idx);Q21=CapacityMatrix(T_out_lower_idx,T_amb_upper_idx);Q22=CapacityMatrix(T_out_upper_idx,T_amb_upper_idx);
        P11=PowerMatrix(T_out_lower_idx,T_amb_lower_idx);P12=PowerMatrix(T_out_upper_idx,T_amb_lower_idx);P21=PowerMatrix(T_out_lower_idx,T_amb_upper_idx);P22=PowerMatrix(T_out_upper_idx,T_amb_upper_idx);
        wx=(T_amb-x1)/(x2-x1);wy=(T_out-y1)/(y2-y1);
        Q_rated=(1-wx)*(1-wy)*Q11+wx*(1-wy)*Q21+(1-wx)*wy*Q12+wx*wy*Q22;P_rated=(1-wx)*(1-wy)*P11+wx*(1-wy)*P21+(1-wx)*wy*P12+wx*wy*P22;
    end
    Q_rated=max(0.2,Q_rated);P_rated=max(0.1,P_rated);
    PLR=min(1,Q_load/Q_rated);PLR_min=0.20;
    if PLR<PLR_min, runtime_fraction=PLR/PLR_min; P_heat=runtime_fraction*(Q_rated*PLR_min); P_el=runtime_fraction*(P_rated*PLR_min*0.94);
    else, part_load_factor=1.0-((1.0-PLR)*0.10); P_heat=Q_rated*PLR; P_el=P_rated*PLR/part_load_factor; end
    if T_amb<10, P_el=P_el*(1.0+max(0,(10-T_amb)*0.01)); end
    if(P_heat-P_el)<=0, P_el=P_heat*0.95; end
    Q_short=max(0,Q_load-P_heat);
end

function [P_heat, P_el, Q_short, T_brine_out] = hpHeatingPartLoad_GSHP_Original_PLM(brine_in, T_out, Q_load, m_dot)
    cp = 4.2;
    if Q_load<=0||brine_in<-5||T_out<25, P_heat=0;P_el=0;Q_short=Q_load;T_brine_out=brine_in;return;end
    brine_in_vec=[0,5,10,15,20];T_out_vec=[30,35,40,45];
    CapacityMatrix=[4.50,4.40,4.30,4.20,4.10;4.35,4.25,4.15,4.05,3.95;4.15,4.05,3.95,3.85,3.75;3.90,3.80,3.70,3.60,3.50];
    PowerMatrix=[1.15,1.12,1.09,1.06,1.03;1.20,1.17,1.14,1.11,1.08;1.25,1.22,1.19,1.16,1.13;1.30,1.27,1.24,1.21,1.18];
    brine_lower_idx=1;for i=1:length(brine_in_vec),if brine_in>=brine_in_vec(i),brine_lower_idx=i;end,end
    if brine_lower_idx==length(brine_in_vec),brine_upper_idx=brine_lower_idx;else,brine_upper_idx=brine_lower_idx+1;end
    T_out_lower_idx=1;for i=1:length(T_out_vec),if T_out>=T_out_vec(i),T_out_lower_idx=i;end,end
    if T_out_lower_idx==length(T_out_vec),T_out_upper_idx=T_out_lower_idx;else,T_out_upper_idx=T_out_lower_idx+1;end
    if brine_lower_idx==brine_upper_idx||T_out_lower_idx==T_out_upper_idx,Q_rated=CapacityMatrix(T_out_lower_idx,brine_lower_idx);P_rated=PowerMatrix(T_out_lower_idx,brine_lower_idx);
    else
        x1=brine_in_vec(brine_lower_idx);x2=brine_in_vec(brine_upper_idx);y1=T_out_vec(T_out_lower_idx);y2=T_out_vec(T_out_upper_idx);
        Q11=CapacityMatrix(T_out_lower_idx,brine_lower_idx);Q12=CapacityMatrix(T_out_upper_idx,brine_lower_idx);Q21=CapacityMatrix(T_out_lower_idx,brine_upper_idx);Q22=CapacityMatrix(T_out_upper_idx,brine_upper_idx);
        P11=PowerMatrix(T_out_lower_idx,brine_lower_idx);P12=PowerMatrix(T_out_upper_idx,brine_lower_idx);P21=PowerMatrix(T_out_lower_idx,brine_upper_idx);P22=PowerMatrix(T_out_upper_idx,brine_upper_idx);
        wx=(brine_in-x1)/(x2-x1);wy=(T_out-y1)/(y2-y1);
        Q_rated=(1-wx)*(1-wy)*Q11+wx*(1-wy)*Q21+(1-wx)*wy*Q12+wx*wy*Q22;P_rated=(1-wx)*(1-wy)*P11+wx*(1-wy)*P21+(1-wx)*wy*P12+wx*wy*P22;
    end
    Q_rated=max(0.1,Q_rated);P_rated=max(0.1,P_rated);
    PLR=min(1,Q_load/Q_rated);PLR_min=0.20;
    if PLR<PLR_min, runtime_fraction=PLR/PLR_min; P_heat=runtime_fraction*(Q_rated*PLR_min); P_el=runtime_fraction*(P_rated*PLR_min*0.90);
    else, part_load_factor=1.0-((1.0-PLR)*0.18); P_heat=Q_rated*PLR; P_el=P_rated*PLR/part_load_factor; end
    Q_evap=P_heat-P_el;
    if Q_evap<=0,P_el=P_heat*0.95;Q_evap=P_heat-P_el;end
    T_brine_out=brine_in-(Q_evap/(m_dot*cp));
    freeze_trigger_temp=0.5;freeze_lockout_temp=-0.5;derating_factor=1.0;
    if brine_in<=freeze_lockout_temp,derating_factor=0.0;
    elseif brine_in<=freeze_trigger_temp,derating_range=freeze_trigger_temp-freeze_lockout_temp;derating_factor=(brine_in-freeze_lockout_temp)/derating_range;end
    derating_factor=min(max(derating_factor,0.0),1.0);
    if derating_factor<1.0
        P_heat=P_heat*derating_factor;P_el=P_el*derating_factor;Q_evap=P_heat-P_el;
        T_brine_out=brine_in-(Q_evap/(m_dot*cp));
    end
    Q_short=max(0,Q_load-P_heat);
end

== matlab function HHP_simulation/GSHP_On//Off ==
  data: u input; y output
function y = fcn(u)
    % Function to check if the ambient temperature is within the range
    % Inputs:
    %   u - Ambient temperature (numeric or part of a structure)
    % Outputs:
    %   y - 1 if the temperature is between 4.9 and -5.3, 0 otherwise

    % Initialize output
    y = 0;

    % Check if input is numeric
    if isnumeric(u)
        % Main logic: check if within range
        if u >= -5.4 && u <= 5
            y = 1;
        end
    % Check if input is a structure
    elseif isstruct(u)
        % Update the field name to match the actual structure
        fieldName = 'Temp'; % Replace with the actual field name
        
        % Ensure the structure has the expected field
        if isfield(u, fieldName)
            temp = u.(fieldName); % Extract the temperature field
            
            % Ensure the extracted value is numeric
            if isnumeric(temp)
                % Main logic: check if within range
                if temp >= -5.4 && temp <= 5
                    y = 1;
                end
            else
                error('The field "%s" must contain numeric data.', fieldName);
            end
        else
            error('The input structure does not have the field "%s".', fieldName);
        end
    else
        % Handle unsupported input types
        error('Input must be either numeric or a structure with a numeric field "%s".', fieldName);
    end
end

== matlab function HHP_simulation/MATLAB Function3 ==
  data: u input; y output
function y = fcn(u)
    % Function to check if the ambient temperature is below 4.9°C
    % Inputs:
    %   u - Ambient temperature (numeric or part of a structure)
    % Outputs:
    %   y - 1 if the temperature is below 4.9°C, 0 otherwise

    % Initialize output
    y = 0;

    % Define the field name (update if needed)
    fieldName = 'Temp'; % Replace with your actual field name if different

    % Check if input is numeric
    if isnumeric(u)
        % Main logic: check if below 4.9°C
        if u < 4.9
            y = 1;
        end
    % Check if input is a structure
    elseif isstruct(u)
        % Ensure the structure has the expected field
        if isfield(u, fieldName)
            temp = u.(fieldName); % Extract the temperature field

            % Ensure the extracted value is numeric
            if isnumeric(temp)
                % Main logic: check if below 4.9°C
                if temp < 4.9
                    y = 1;
                end
            else
                error('The field "%s" must contain numeric data.', fieldName);
            end
        else
            error('The input structure does not have the field "%s".', fieldName);
        end
    else
        % Handle unsupported input types
        error('Input must be either numeric or a structure with a numeric field "%s".', fieldName);
    end
end

== matlab function HHP_simulation/PSHP_On//Off ==
  data: u input; y output
function y = fcn(u)
   % Function to check if the ambient temperature is below -5.4°C
   % Inputs:
   %   u - Ambient temperature (numeric or part of a structure)
   % Outputs:
   %   y - 1 if the temperature is below -5.4°C, 0 otherwise
   % Initialize output
   y = 0;
   if isnumeric(u)
       % Main logic: check if below -5.4°C
       if u <= -5.4
           y = 1;
       end
   % Check if input is a structure
   elseif isstruct(u)
       % Ensure the structure has the expected field
       if isfield(u, fieldName)
           temp = u.(fieldName); % Extract the temperature field
           % Ensure the extracted value is numeric
           if isnumeric(temp)
               % Main logic: check if below -5.4°C
               if temp <= -5.4
                   y = 1;
               end
           else
               error('The field "%s" must contain numeric data.', fieldName);
           end
       else
           error('The input structure does not have the field "%s".', fieldName);
       end
   else
       % Handle unsupported input types
       error('Input must be either numeric or a structure with a numeric field "%s".', fieldName);
   end
end
